simulink model "PNG"  (R2026a)
settings: Solver=FixedStepDiscrete  StopTime=1e-3  FixedStep=1e-5

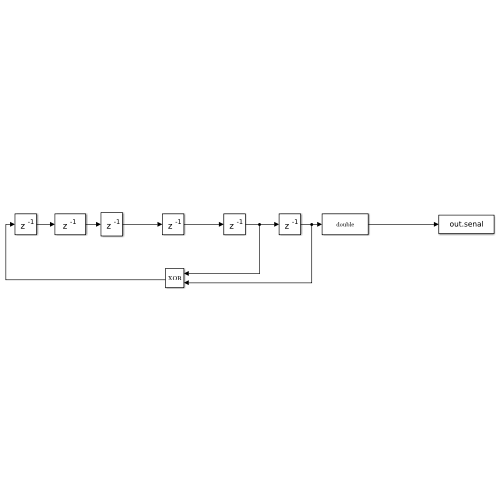
[thumbnail: Simulink's stored preview of the top-level diagram]
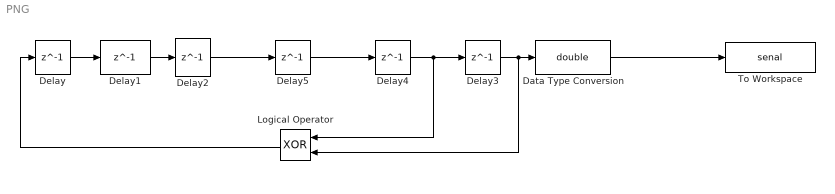
== system PNG ==
  Data Type Conversion : DataTypeConversion  OutDataTypeStr=double  SaturateOnIntegerOverflow=off  RndMeth=Floor
  Delay : Delay  DelayLength=1  InitialCondition=1
  Delay1 : Delay  DelayLength=1
  Delay2 : Delay  DelayLength=1  InitialCondition=1
  Delay3 : Delay  DelayLength=1  InitialCondition=1
  Delay4 : Delay  DelayLength=1
  Delay5 : Delay  DelayLength=1
  Logical Operator : Logic  Operator=XOR  AllPortsSameDT=off  OutDataTypeStr=boolean
  To Workspace : ToWorkspace  VariableName=senal  SampleTime=-1
  wires:
  Delay4/1 -> Logical Operator/1, Delay3/1
  Delay1/1 -> Delay2/1
  Delay/1 -> Delay1/1
  Delay2/1 -> Delay5/1
  Delay5/1 -> Delay4/1
  Delay3/1 -> Logical Operator/2, Data Type Conversion/1
  Logical Operator/1 -> Delay/1
  Data Type Conversion/1 -> To Workspace/1
